simulink model "OnePhaseInductionMotor"  (R2017b)
settings: Solver=VariableStepAuto  StartTime=0.0  StopTime=0.2  MaxStep=1e-4  RelTol=1e-3
undefined symbols (not defined in the file or in its folder): i
libraries: powerlib x5, powerlib_meascontrol x1
settings Model: Creator=Makdissi  LastModifiedBy=Makdissi

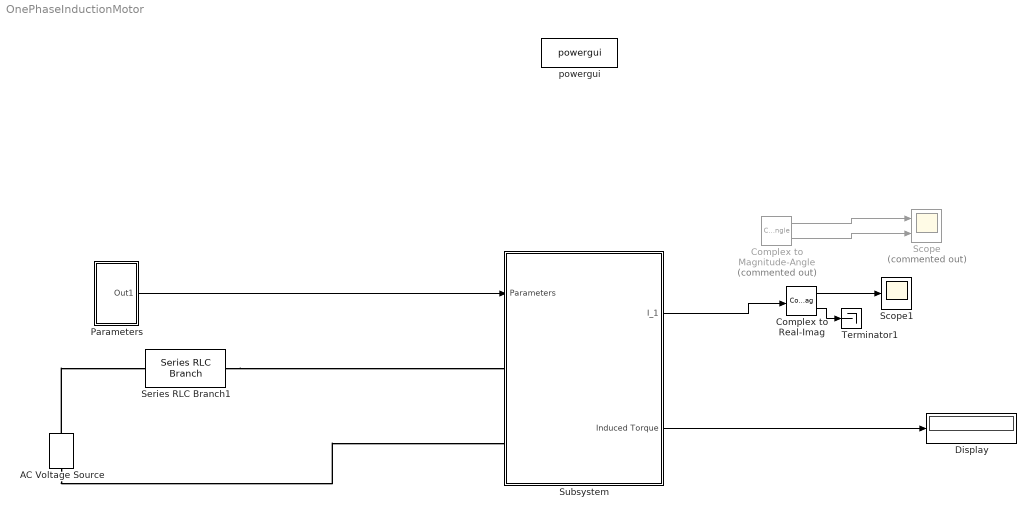
== system OnePhaseInductionMotor ==
  AC Voltage Source : powerlib/Electrical Sources/AC Voltage Source  Amplitude=266  Phase=0  Frequency=60  SampleTime=0  Measurements=None  BusType=swing  Pref=10e3  Qref=0  Qmin=-inf  Qmax=+inf
  Complex to Magnitude-Angle : ComplexToMagnitudeAngle  Commented=on
  Complex to Real-Imag : ComplexToRealImag
  Display : Display
  Parameters : Subsystem
  Scope : Scope  Commented=on  NumInputPorts=2
  Scope1 : Scope
  Series RLC Branch1 : powerlib/Elements/Series RLC Branch  LConnTagsString=__new0  RConnTagsString=__new0  BranchType=R  Resistance=0.1  Inductance=1e-3  SetiL0=off  InitialCurrent=0  Capacitance=1e-6  Setx0=off  InitialVoltage=0  Measurements=None
  Subsystem : Subsystem
  Terminator1 : Terminator
  powergui : powerlib/powergui  Priority=1  SimulationMode=Continuous  SampleTime=50e-6  frequency=60  Iterations=50  frequencyindice=60  Pbase=100e6  ErrMax=1e-4  UnitsV=kV  UnitsW=MW  buscounter=0  FunctionMessages=off  echomessages=off  EnableUseOfTLC=off  CurrentSourceSwitches=off  DisableSnubberDevices=off  DisableRonSwitches=off  DisableVfSwitches=off  DisplayEquations=off  SolverType=Tustin/Backward Euler (TBE)  Interpol=off  ExternalGateDelay=off  methode=off  Ts=100  x0status=blocks  SPID=on  SwTol=0  HookPort=off  RestoreLinks=warning  ResistiveCurrentMeasurement=off  Frange=[0:2:500]  Ylog=off  Xlog=on  ShowGrid=off  save=off  variable=ZData  structure=0  ZoomFFT=off  StartTime=0.0  cycles=1  DisplayStyle=1  fundamental=60  FreqAxis=off  MaxFrequency=1000  frequencyindicesteady=1  RmsSteady=1  display=off
  wires:
  Parameters/1(Out1) -> Subsystem/1(Parameters)
  Subsystem/1(I_1) -> Complex to Real-Imag/1
  Complex to Magnitude-Angle/1 -> Scope/1
  Complex to Magnitude-Angle/2 -> Scope/2
  Complex to Real-Imag/1 -> Scope1/1
  Complex to Real-Imag/2 -> Terminator1/1
  Subsystem/2(Induced Torque) -> Display/1
  connections:
  Series RLC Branch1/RConn1 -- Subsystem/LConn1
  AC Voltage Source/LConn1 -- Subsystem/LConn2
  AC Voltage Source/RConn1 -- Series RLC Branch1/LConn1

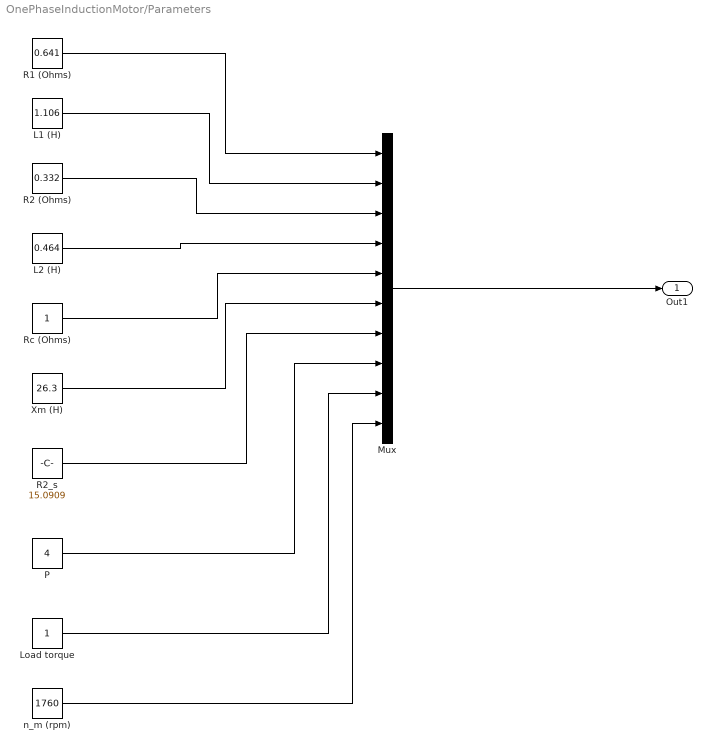
== system OnePhaseInductionMotor/Parameters ==
  L1 (H) : Constant  Value=1.106
  L2 (H) : Constant  Value=0.464
  Load torque : Constant
  Mux : Mux  Inputs=10
  P : Constant  Value=4
  R1 (Ohms) : Constant  Value=0.641
  R2 (Ohms) : Constant  Value=0.332
  R2_s : Constant  Value=15.0909
  Rc (Ohms) : Constant
  Xm (H) : Constant  Value=26.3
  n_m (rpm) : Constant  Value=1760
  Out1 : Outport
  wires:
  Mux/1 -> Out1/1
  L1 (H)/1 -> Mux/2
  R1 (Ohms)/1 -> Mux/1
  R2 (Ohms)/1 -> Mux/3
  Xm (H)/1 -> Mux/6
  R2_s/1 -> Mux/7
  P/1 -> Mux/8
  Rc (Ohms)/1 -> Mux/5
  L2 (H)/1 -> Mux/4
  Load torque/1 -> Mux/9
  n_m (rpm)/1 -> Mux/10

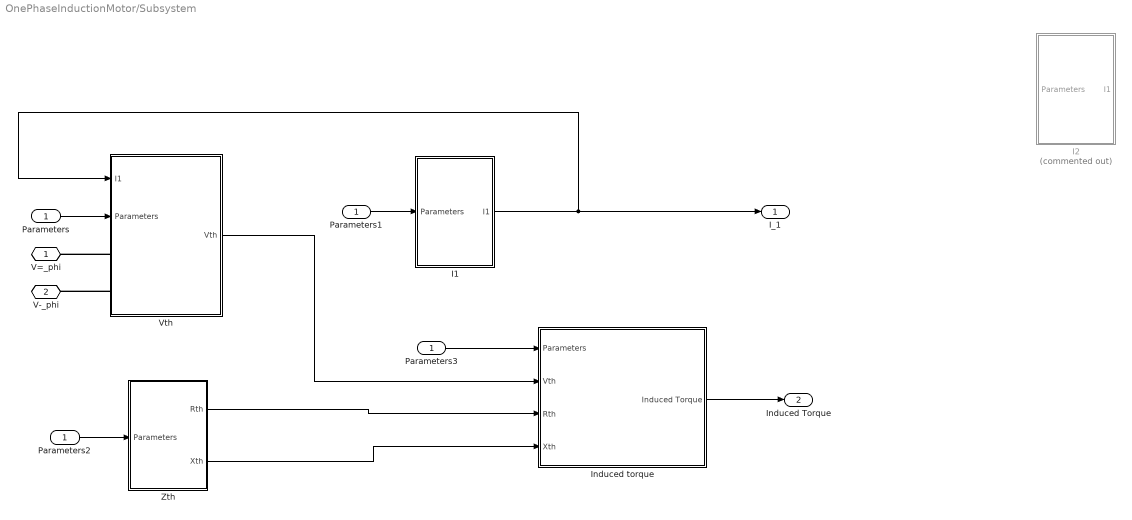
== system OnePhaseInductionMotor/Subsystem ==
  Parameters : Inport
  I1 : Subsystem
  I2 : Subsystem  Commented=on
  Induced torque : Subsystem
  Parameters1 : InportShadow
  Parameters2 : InportShadow
  Parameters3 : InportShadow
  Vth : Subsystem
  Zth : Subsystem
  V=_phi : PMIOPort  Port=1  Side=Left
  V-_phi : PMIOPort  Port=2  Side=Left
  I_1 : Outport
  Induced Torque : Outport  Port=2
  wires:
  Parameters/1 -> Vth/2(Parameters)
  I1/1(I1) -> Vth/1(I1), I_1/1
  Parameters1/1 -> I1/1(Parameters)
  Parameters2/1 -> Zth/1(Parameters)
  Parameters3/1 -> Induced torque/1(Parameters)
  Induced torque/1(Induced Torque) -> Induced Torque/1
  Zth/1(Rth) -> Induced torque/3(Rth)
  Zth/2(Xth) -> Induced torque/4(Xth)
  Vth/1(Vth) -> Induced torque/2(Vth)
  connections:
  Vth/LConn2 -- V-_phi/RConn1
  Vth/LConn1 -- V=_phi/RConn1

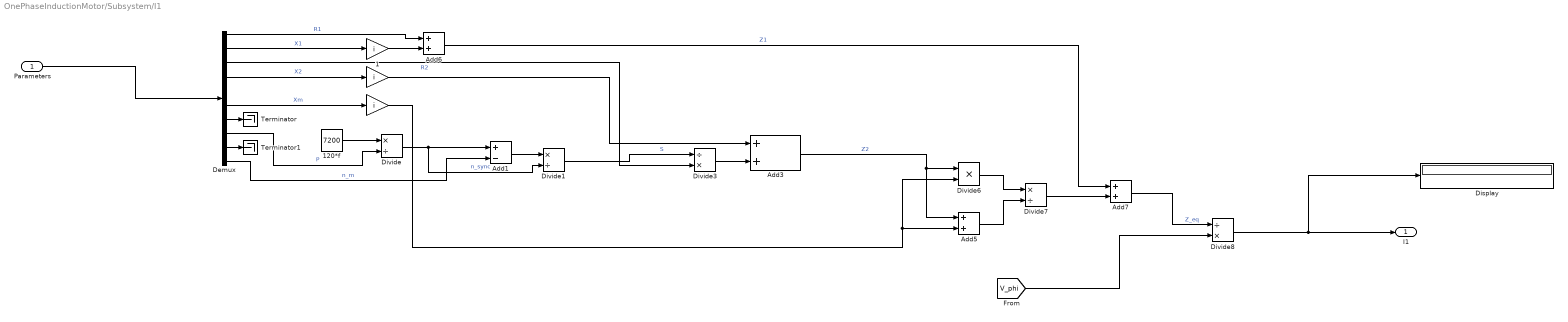
== system OnePhaseInductionMotor/Subsystem/I1 ==
  Parameters : Inport
  " " : Gain  Gain=i
  " " : Gain  Gain=i
  " 1" : Gain  Gain=i
  120*f : Constant  Value=7200
  Add1 : Sum  Inputs=+-
  Add{3,5..7} (4 alike) : Sum
  Demux : Demux  Outputs=10
  Display : Display
  Divide : Product  Inputs=*/
  Divide1 : Product  Inputs=*/
  Divide3 : Product  Inputs=/*
  Divide6 : Product  Inputs=**
  Divide7 : Product  Inputs=*/
  Divide8 : Product  Inputs=/*
  Terminator : Terminator
  Terminator1 : Terminator
  I1 : Outport
  wires:
  Parameters/1 -> Demux/1
  120*f/1 -> Divide/1
  Demux/8 -> Divide/2  "P"
  Divide/1 -> Divide1/2, Add1/1  "n_sync"
  Demux/10 -> Add1/2  "n_m"
  Add1/1 -> Divide1/1
  Divide1/1 -> Divide3/1  "S"
  Demux/3 -> Divide3/2  "R2"
  Demux/4 -> " "/1  "X2"
  " "/1 -> Add3/1
  Demux/6 -> " "/1  "Xm"
  " "/1 -> Divide6/2, Add5/2
  Add3/1 -> Add5/1, Divide6/1  "Z2"
  Divide6/1 -> Divide7/1
  Add5/1 -> Divide7/2
  Demux/2 -> " 1"/1  "X1"
  " 1"/1 -> Add6/2
  Demux/1 -> Add6/1  "R1"
  Add6/1 -> Add7/1  "Z1"
  Divide7/1 -> Add7/2
  [V_phi] -> Divide8/2
  Add7/1 -> Divide8/1  "Z_eq"
  Divide8/1 -> Display/1, I1/1
  Demux/7 -> Terminator/1
  Demux/9 -> Terminator1/1
  Divide3/1 -> Add3/2

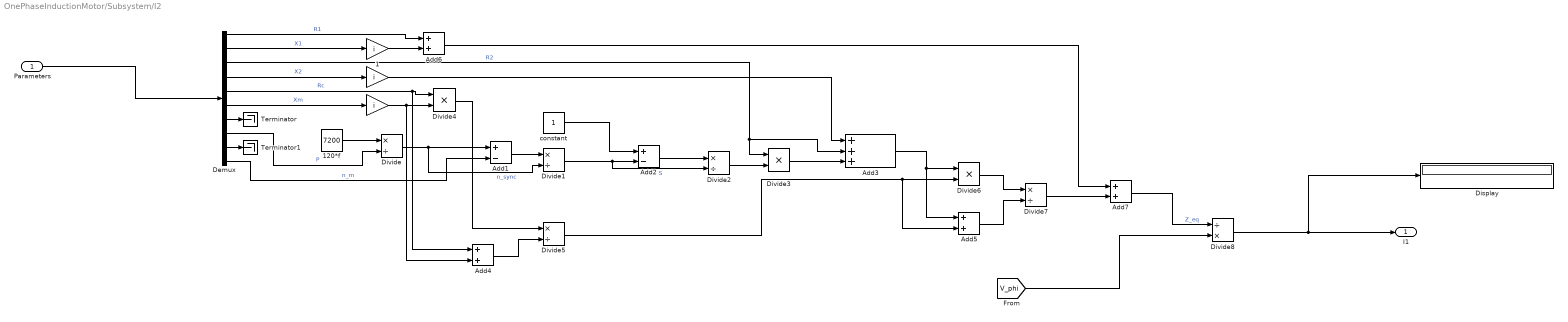
== system OnePhaseInductionMotor/Subsystem/I2 ==
  Parameters : Inport
  " " : Gain  Gain=i
  " " : Gain  Gain=i
  " 1" : Gain  Gain=i
  120*f : Constant  Value=7200
  Add1 : Sum  Inputs=+-
  Add2 : Sum  Inputs=+-
  Add3 : Sum  Inputs=+++
  Add{4..7} (4 alike) : Sum
  Demux : Demux  Outputs=10
  Display : Display
  Divide{,1..2,5,7} (5 alike) : Product  Inputs=*/
  Divide3 : Product  Inputs=**
  Divide4 : Product  Inputs=**
  Divide6 : Product  Inputs=**
  Divide8 : Product  Inputs=/*
  Terminator : Terminator
  Terminator1 : Terminator
  constant : Constant
  I1 : Outport
  wires:
  Demux/9 -> Terminator1/1
  Demux/7 -> Terminator/1
  Divide8/1 -> I1/1, Display/1
  Add7/1 -> Divide8/1  "Z_eq"
  [V_phi] -> Divide8/2
  Divide7/1 -> Add7/2
  Add6/1 -> Add7/1
  Demux/1 -> Add6/1  "R1"
  " 1"/1 -> Add6/2
  Demux/2 -> " 1"/1  "X1"
  Add5/1 -> Divide7/2
  Divide6/1 -> Divide7/1
  Add3/1 -> Divide6/1, Add5/1
  Divide5/1 -> Divide6/2, Add5/2
  Add4/1 -> Divide5/2
  Divide4/1 -> Divide5/1
  " "/1 -> Divide4/2, Add4/2
  Demux/5 -> Divide4/1, Add4/1  "Rc"
  Demux/6 -> " "/1  "Xm"
  " "/1 -> Add3/1
  Demux/4 -> " "/1  "X2"
  Divide3/1 -> Add3/3
  Divide2/1 -> Divide3/2
  Demux/3 -> Divide3/1, Add3/2  "R2"
  Add2/1 -> Divide2/1
  Divide1/1 -> Add2/2, Divide2/2  "S"
  constant/1 -> Add2/1
  Add1/1 -> Divide1/1
  Demux/10 -> Add1/2  "n_m"
  Divide/1 -> Add1/1, Divide1/2  "n_sync"
  Demux/8 -> Divide/2  "P"
  120*f/1 -> Divide/1
  Parameters/1 -> Demux/1

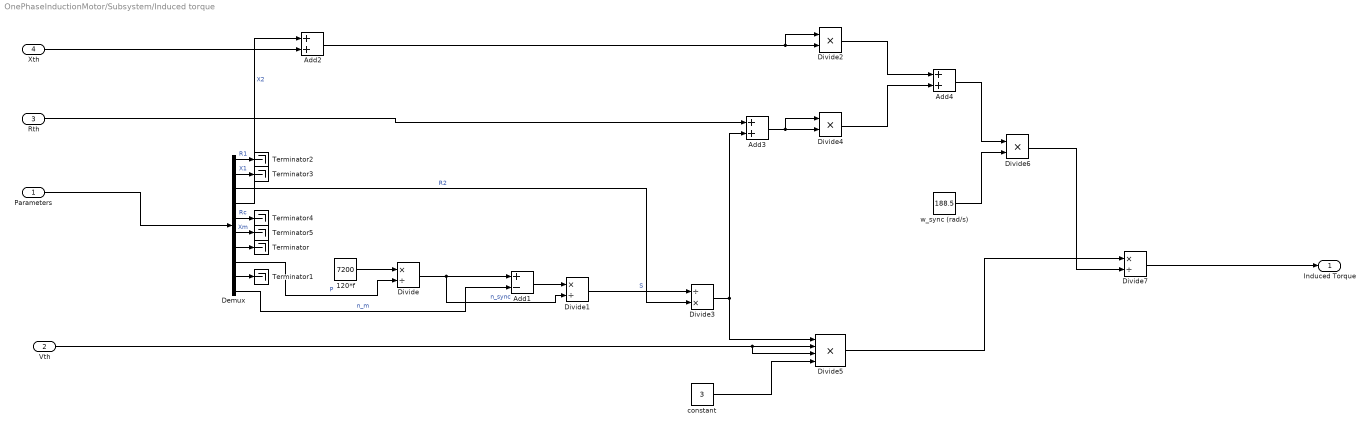
== system OnePhaseInductionMotor/Subsystem/Induced torque ==
  Parameters : Inport
  Vth : Inport  Port=2
  Rth : Inport  Port=3
  Xth : Inport  Port=4
  120*f : Constant  Value=7200
  Add1 : Sum  Inputs=+-
  Add2 : Sum
  Add3 : Sum
  Add4 : Sum
  Demux : Demux  Outputs=10
  Divide : Product  Inputs=*/
  Divide1 : Product  Inputs=*/
  Divide2 : Product  Inputs=**
  Divide3 : Product  Inputs=/*
  Divide4 : Product  Inputs=**
  Divide5 : Product  Inputs=****
  Divide6 : Product  Inputs=**
  Divide7 : Product  Inputs=*/
  Terminator{,1..5} (6 alike) : Terminator
  constant : Constant  Value=3
  w_sync (rad/s) : Constant  Value=188.5
  Induced Torque : Outport
  wires:
  Divide3/1 -> Divide5/1, Add3/2
  Demux/9 -> Terminator1/1
  Demux/7 -> Terminator/1
  Divide7/1 -> Induced Torque/1
  Demux/4 -> Add2/1  "X2"
  Demux/3 -> Divide3/2  "R2"
  Divide1/1 -> Divide3/1  "S"
  Add1/1 -> Divide1/1
  Demux/10 -> Add1/2  "n_m"
  Divide/1 -> Add1/1, Divide1/2  "n_sync"
  Demux/8 -> Divide/2  "P"
  120*f/1 -> Divide/1
  Parameters/1 -> Demux/1
  Demux/1 -> Terminator2/1  "R1"
  Demux/2 -> Terminator3/1  "X1"
  Demux/5 -> Terminator4/1  "Rc"
  Demux/6 -> Terminator5/1  "Xm"
  Xth/1 -> Add2/2
  Add2/1 -> Divide2/1, Divide2/2
  Add3/1 -> Divide4/1, Divide4/2
  Rth/1 -> Add3/1
  Divide2/1 -> Add4/1
  Divide4/1 -> Add4/2
  Add4/1 -> Divide6/1
  w_sync (rad/s)/1 -> Divide6/2
  constant/1 -> Divide5/4
  Divide5/1 -> Divide7/1
  Divide6/1 -> Divide7/2
  Vth/1 -> Divide5/3, Divide5/2

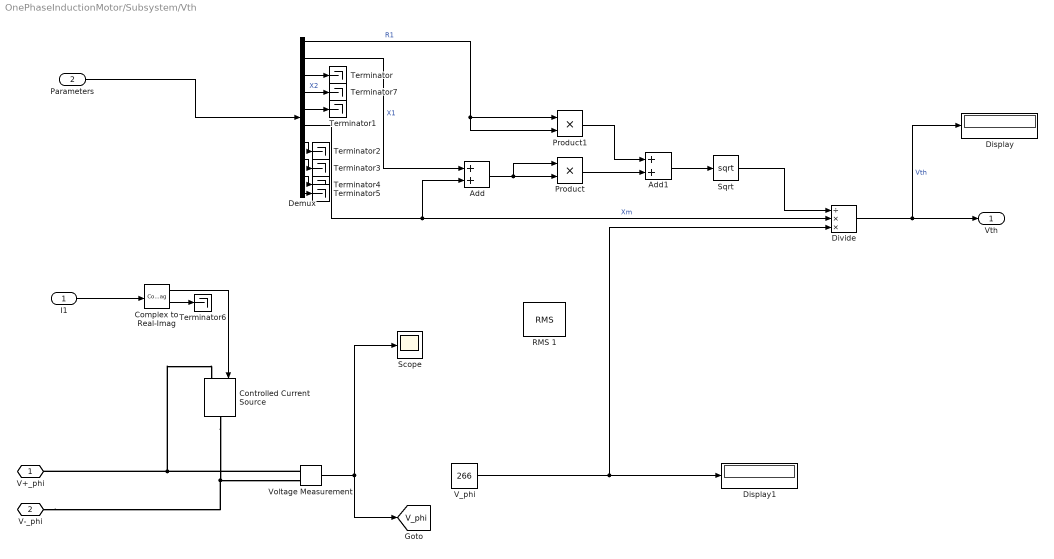
== system OnePhaseInductionMotor/Subsystem/Vth ==
  I1 : Inport
  Parameters : Inport  Port=2
  Add : Sum
  Add1 : Sum
  Complex to Real-Imag : ComplexToRealImag
  Controlled Current Source : powerlib/Electrical Sources/Controlled Current Source  Initialize=on  Source_Type=AC  Amplitude=0  Phase=0  Frequency=0  Measurements=Current
  Demux : Demux  Outputs=10
  Display : Display
  Display1 : Display
  Divide : Product  Inputs=/**
  Product : Product
  Product1 : Product
  RMS 1 : powerlib_meascontrol/Measurements/RMS  TrueRMS=on  Freq=60  RMSInit=188.1  Ts=0.000002
  Scope : Scope
  Sqrt : Sqrt  SaturateOnIntegerOverflow=on
  Terminator{,1..7} (8 alike) : Terminator
  V_phi : Constant  Value=266
  Voltage Measurement : powerlib/Measurements/Voltage Measurement  PhasorSimulation=off  OutputType=Complex  PSBequivalent=0
  V+_phi : PMIOPort  Port=1  Side=Left
  V-_phi : PMIOPort  Port=2  Side=Left
  Vth : Outport
  tag scope: V_phi=global
  wires:
  Parameters/1 -> Demux/1
  Demux/2 -> Add/1  "X1"
  Demux/6 -> Add/2, Divide/2  "Xm"
  Add/1 -> Product/1, Product/2
  Product/1 -> Add1/2
  Demux/1 -> Product1/2, Product1/1  "R1"
  Product1/1 -> Add1/1
  Add1/1 -> Sqrt/1
  Sqrt/1 -> Divide/1
  Divide/1 -> Display/1, Vth/1  "Vth"
  Demux/3 -> Terminator/1
  Demux/5 -> Terminator1/1
  Demux/7 -> Terminator2/1
  Demux/8 -> Terminator3/1
  Demux/9 -> Terminator4/1
  Demux/10 -> Terminator5/1
  Complex to Real-Imag/1 -> Controlled Current Source/1
  Complex to Real-Imag/2 -> Terminator6/1
  I1/1 -> Complex to Real-Imag/1
  Voltage Measurement/1 -> [V_phi], Scope/1
  Demux/4 -> Terminator7/1  "X2"
  V_phi/1 -> Divide/3, Display1/1
  connections:
  Voltage Measurement/LConn1 -- V+_phi/RConn1 -- Controlled Current Source/LConn1
  V-_phi/RConn1 -- Voltage Measurement/LConn2 -- Controlled Current Source/RConn1

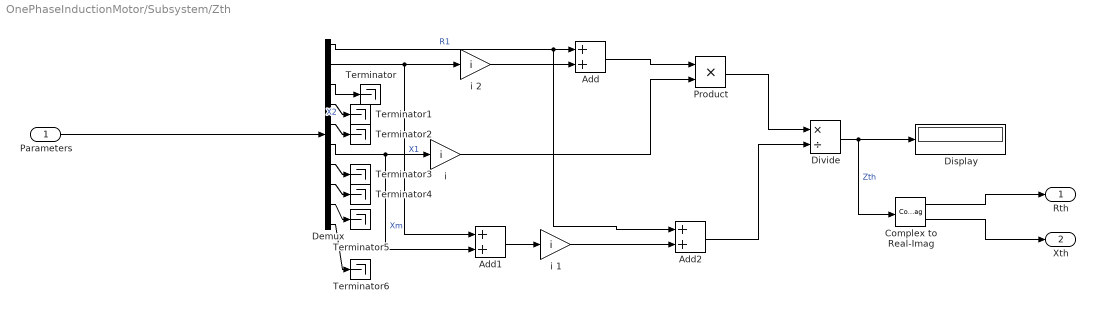
== system OnePhaseInductionMotor/Subsystem/Zth ==
  Parameters : Inport
  Add : Sum
  Add1 : Sum
  Add2 : Sum
  Complex to Real-Imag : ComplexToRealImag
  Demux : Demux  Outputs=10
  Display : Display
  Divide : Product  Inputs=*/
  Product : Product
  Terminator{,1..6} (7 alike) : Terminator
  "i " : Gain  Gain=i
  i 1 : Gain  Gain=i
  i 2 : Gain  Gain=i
  Rth : Outport
  Xth : Outport  Port=2
  wires:
  Parameters/1 -> Demux/1
  Demux/1 -> Add2/1, Add/1  "R1"
  Demux/6 -> Add1/2, "i "/1  "Xm"
  Demux/2 -> Add1/1, i 2/1  "X1"
  Add/1 -> Product/1
  Add1/1 -> i 1/1
  i 1/1 -> Add2/2
  Add2/1 -> Divide/2
  Product/1 -> Divide/1
  Divide/1 -> Complex to Real-Imag/1, Display/1  "Zth"
  Demux/3 -> Terminator/1
  Demux/4 -> Terminator1/1  "X2"
  Demux/5 -> Terminator2/1
  Demux/7 -> Terminator3/1
  Demux/8 -> Terminator4/1
  Demux/9 -> Terminator5/1
  Demux/10 -> Terminator6/1
  "i "/1 -> Product/2
  i 2/1 -> Add/2
  Complex to Real-Imag/1 -> Rth/1
  Complex to Real-Imag/2 -> Xth/1
